simulink model "LoadFlow116BusNetwork_original"  (R2024a)
settings: Solver=FixedStepDiscrete  StartTime=0.0  StopTime=4.5  FixedStep=75e-6  RelTol=1e-3  EnableMultiTasking=on
undefined symbols (not defined in the file or in its folder): D1, D11, Delta
libraries: spsSeriesRLCBranchLib x164, spsLoadFlowBusLib x116, spsDistributedParametersLineLib x79, spsThreePhaseSeriesRLCLoadLib x60, spsThreePhaseTransformerTwoWindingsLib x52, spsThreePhaseParallelRLCLoadLib x44, spsThreePhaseVIMeasurementLib x44, spsSynchronousMachinepuStandardLib x28, spsExcitationSystemLib x28, spsHydraulicTurbineandGovernorLib x28, spsGenericPowerSystemStabilizerLib x28, spsMultiBandPowerSystemStabilizerLib x28
(part 6 of 15)

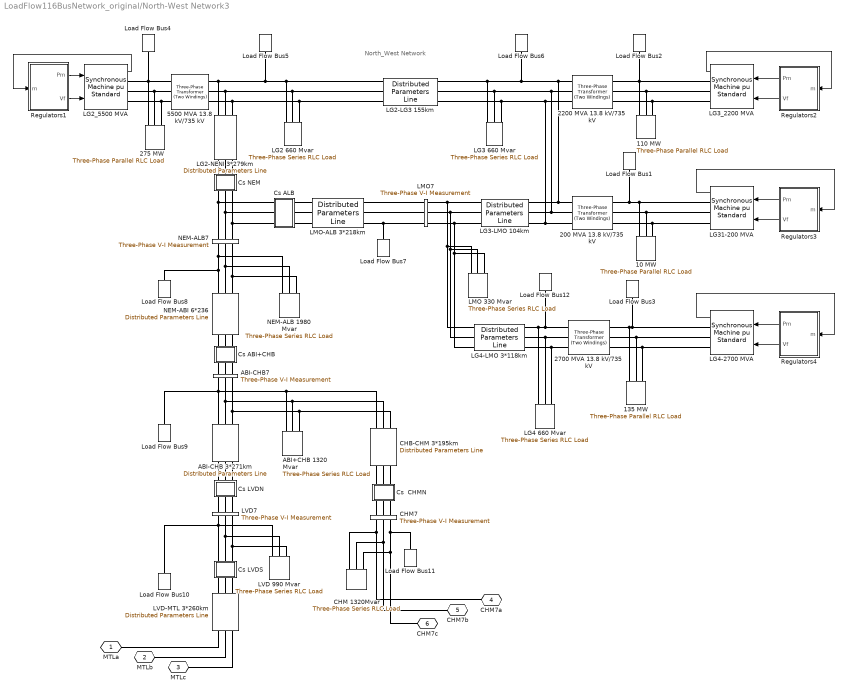
== system LoadFlow116BusNetwork_original/North-West Network3 ==
  note: North_West Network
  10 MW : spsThreePhaseParallelRLCLoadLib/Three-Phase Parallel RLC Load  LConnTagsString=A|B|C  Configuration=Y (grounded)  NominalVoltage=(13800)*1  Vabc=[1e3 1e3 1e3]  Vabcp=[1e3 1e3 1e3]  NominalFrequency=60  UnbalancedPower=off  ActivePower=10000000  InductivePower=0  CapacitivePower=0  Pabc=[10e3 9e3 11e3]  QLabc=[100 90 110]  QCabc=[100 90 110]  Pabcp=[10e3 9e3 11e3]  QLabcp=[100 90 110]  QCabcp=[100 90 110]  Measurements=None  LoadType=constant PQ
  110 MW : spsThreePhaseParallelRLCLoadLib/Three-Phase Parallel RLC Load  LConnTagsString=A|B|C  Configuration=Y (grounded)  NominalVoltage=(13800)*1  Vabc=[1e3 1e3 1e3]  Vabcp=[1e3 1e3 1e3]  NominalFrequency=60  UnbalancedPower=off  ActivePower=110000000  InductivePower=0  CapacitivePower=0  Pabc=[10e3 9e3 11e3]  QLabc=[100 90 110]  QCabc=[100 90 110]  Pabcp=[10e3 9e3 11e3]  QLabcp=[100 90 110]  QCabcp=[100 90 110]  Measurements=None  LoadType=constant PQ
  135 MW : spsThreePhaseParallelRLCLoadLib/Three-Phase Parallel RLC Load  LConnTagsString=A|B|C  Configuration=Y (grounded)  NominalVoltage=(13800)*1  Vabc=[1e3 1e3 1e3]  Vabcp=[1e3 1e3 1e3]  NominalFrequency=60  UnbalancedPower=off  ActivePower=135000000  InductivePower=0  CapacitivePower=0  Pabc=[10e3 9e3 11e3]  QLabc=[100 90 110]  QCabc=[100 90 110]  Pabcp=[10e3 9e3 11e3]  QLabcp=[100 90 110]  QCabcp=[100 90 110]  Measurements=None  LoadType=constant PQ
  200 MVA 13.8 kV/735 kV : spsThreePhaseTransformerTwoWindingsLib/Three-Phase Transformer (Two Windings)  Winding1Connection=Delta (D1)  Winding2Connection=Yg  CoreType=Three single-phase transformers  SetSaturation=off  Hysteresis=off  DataFile='basic_model'  SetInitialFlux=off  Measurements=None  UNITS=pu  NominalPower=[ 200e6 60 ]  Winding1="[ 13.8e3 0.002  0.0]"  Winding2=[ 735e3 0.002 0.12]  Rm=500  Lm=500  L0=0.5  Saturation="[ 0,0  ;  0.005,1.2  ;  1.0,1.4 ]"  InitialFluxes=[ 0.8 , -0.8 , 0.7 ]  BreakLoop=off  DiscreteSolver=Trapezoidal iterative  DataType=off  TransfoNumber=0
  2200 MVA 13.8 kV/735 kV : spsThreePhaseTransformerTwoWindingsLib/Three-Phase Transformer (Two Windings)  Winding1Connection=Delta (D1)  Winding2Connection=Yg  CoreType=Three single-phase transformers  SetSaturation=off  Hysteresis=off  DataFile='basic_model'  SetInitialFlux=off  Measurements=None  UNITS=pu  NominalPower=[ 2200e6 60 ]  Winding1="[ 13.8e3 0.002  0.0]"  Winding2=[ 735e3 0.002 0.12]  Rm=500  Lm=500  L0=0.5  Saturation="[ 0,0  ;  0.005,1.2  ;  1.0,1.4 ]"  InitialFluxes=[ 0.8 , -0.8 , 0.7 ]  BreakLoop=off  DiscreteSolver=Trapezoidal iterative  DataType=off  TransfoNumber=0
  2700 MVA 13.8 kV/735 kV : spsThreePhaseTransformerTwoWindingsLib/Three-Phase Transformer (Two Windings)  Winding1Connection=Delta (D1)  Winding2Connection=Yg  CoreType=Three single-phase transformers  SetSaturation=off  Hysteresis=off  DataFile='basic_model'  SetInitialFlux=off  Measurements=None  UNITS=pu  NominalPower=[ 2700e6 60 ]  Winding1="[ 13.8e3 0.002  0.0]"  Winding2=[ 735e3 0.002 0.12]  Rm=500  Lm=500  L0=0.5  Saturation="[ 0,0  ;  0.005,1.2  ;  1.0,1.4 ]"  InitialFluxes=[ 0.8 , -0.8 , 0.7 ]  BreakLoop=off  DiscreteSolver=Trapezoidal iterative  DataType=off  TransfoNumber=0
  275 MW : spsThreePhaseParallelRLCLoadLib/Three-Phase Parallel RLC Load  LConnTagsString=A|B|C  Configuration=Y (grounded)  NominalVoltage=(13800)*1  Vabc=[1e3 1e3 1e3]  Vabcp=[1e3 1e3 1e3]  NominalFrequency=60  UnbalancedPower=off  ActivePower=275000000  InductivePower=0  CapacitivePower=0  Pabc=[10e3 9e3 11e3]  QLabc=[100 90 110]  QCabc=[100 90 110]  Pabcp=[10e3 9e3 11e3]  QLabcp=[100 90 110]  QCabcp=[100 90 110]  Measurements=None  LoadType=constant PQ
  5500 MVA 13.8 kV/735 kV : spsThreePhaseTransformerTwoWindingsLib/Three-Phase Transformer (Two Windings)  Winding1Connection=Delta (D1)  Winding2Connection=Yg  CoreType=Three single-phase transformers  SetSaturation=off  Hysteresis=off  DataFile='basic_model'  SetInitialFlux=off  Measurements=None  UNITS=pu  NominalPower=[ 5500e6 60 ]  Winding1="[ 13.8e3 0.002  0.0]"  Winding2=[ 735e3 0.002 0.12]  Rm=500  Lm=500  L0=0.5  Saturation="[ 0,0  ;  0.005,1.2  ;  1.0,1.4 ]"  InitialFluxes=[ 0.8 , -0.8 , 0.7 ]  BreakLoop=off  DiscreteSolver=Trapezoidal iterative  DataType=off  TransfoNumber=0
  ABI+CHB 1320 Mvar : spsThreePhaseSeriesRLCLoadLib/Three-Phase Series RLC Load  LConnTagsString=A|B|C  Configuration=Y (grounded)  NominalVoltage=735e3  Vabc=[1e3 1e3 1e3]  Vabcp=[1e3 1e3 1e3]  NominalFrequency=60  UnbalancedPower=off  ActivePower=4400000  InductivePower=1320e6  CapacitivePower=0  Pabc=[10e3 9e3 11e3]  QLabc=[100 90 110]  QCabc=[100 90 110]  Pabcp=[10e3 9e3 11e3]  QLabcp=[100 90 110]  QCabcp=[100 90 110]  Measurements=None  LoadType=constant Z
  ABI-CHB 3*271km : spsDistributedParametersLineLib/Distributed Parameters Line  Phases=3  Length=271  Frequency=60  Resistance="[0.01273  0.3864]/3"  Inductance="[0.9337e-3  4.1264e-3]/3"  Capacitance=[12.74e-9 7.751e-9]*3  x1=[-0.001575 1.61368784010764e-08 -103484.456536196 -819305.84711539;-0.0015 1.60869587384057e-08 -80280.8596538857 -821903.919579448;-0.001425 1.60241794070583e-08 -57013.0874807064 -823844.974625746;-0.00135 1.5948590591871e-08 -33699.7399177245 -825127.460604578;-0.001275 1.58602527173862e-08 -10359.4532982758 -825750.352316277;-0.0012 1.57592363995491e-08 12989.1145096347 -825713.151830738;-0.001125 1.56456223892586e-08 36327.2990181464 -825015.88888546;-0.00105 1.55195015078162e-08 59636.4440396491 -823659.120861774;-0.000975 1.53809745743248e-08 82897.9166002548 -821643.932339278;-0.0009 1.52301523250955e-08 106093.121834711 -818971.934228844;-0.000825 1.50671553251267e-08 129203.517850851 -815645.262484878;-0.00075 1.48921138717261e-08 152210.630551702 -811666.576397873;-0.000675 1.47051678903535e-08 175096.068403391 -807039.05646861;-0.0006 1.45064668227659e-08 197841.537137057 -801766.401865718;-0.000525 1.42961695075566e-08 220428.854373013 -795852.827468612;-0.00045 1.40744440531817e-08 242839.964155458 -789303.060498184;-0.000375 1.38414677035769e-08 265056.951386133 -782122.336737935;-0.0003 1.35974266964714e-08 287062.056145378 -774316.396348571;-0.000225 1.33425161145124e-08 308837.687889136 -765891.479279405;-0.00015 1.30769397293187e-08 330366.439510571 -756854.320280235;-7.5e-05 1.28009098385893e-08 351631.101255038 -747212.143517692]  x2=[-0.001575 3.62536968240975e-08 -329701.158011595 -748762.187115594;-0.0015 3.6150290335032e-08 -308401.441010007 -757783.743021083;-0.001425 3.60179858569907e-08 -286855.192615176 -766199.538196882;-0.00135 3.5856889152149e-08 -265079.636568401 -774002.845185091;-0.001275 3.56671289987478e-08 -243092.179916007 -781187.426141501;-0.0012 3.54488570881504e-08 -220910.399094423 -787747.537822021;-0.001125 3.52022479035825e-08 -198552.025879845 -793677.936173748;-0.00105 3.49274985806529e-08 -176034.933213728 -798973.880526977;-0.000975 3.46248287497665e-08 -153377.120915423 -803631.137384824;-0.0009 3.42944803605553e-08 -130596.701293408 -807645.983807413;-0.000825 3.39367174884669e-08 -107711.884666575 -811015.210387945;-0.00075 3.35518261236675e-08 -84740.9648071874 -813736.123818242;-0.000675 3.31401139424249e-08 -61702.3043171127 -815806.549041739;-0.0006 3.27019100611576e-08 -38614.3199490438 -817224.83099219;-0.000525 3.22375647733433e-08 -15495.4678844266 -817989.835916705;-0.00045 3.17474492695005e-08 7635.77102012883 -818100.952282053;-0.000375 3.1231955340464e-08 30760.906006162 -817558.091263511;-0.0003 3.06914950641932e-08 53861.4511945915 -816361.686815871;-0.000225 3.01265004763637e-08 76918.9403630438 -814512.695326543;-0.00015 2.95374232250043e-08 99914.9417074692 -812012.594851034;-7.5e-05 2.89247342094566e-08 122831.072576244 -808863.383931409]  x3=[-0.001575 1.03818529884453e-10 -747.84143391774 -1501.46113433694;-0.0015 1.07871324417376e-10 -705.095036948362 -1522.00231179514;-0.001425 1.11837888264047e-10 -661.784997794763 -1541.3268238927;-0.00135 1.15715050614017e-10 -617.945937839577 -1559.41922291034;-0.001275 1.19499712123026e-10 -573.612901356573 -1576.2650460611;-0.0012 1.2318884739057e-10 -528.821327496795 -1591.8508270517;-0.001125 1.26779507378363e-10 -483.607021959054 -1606.16410684729;-0.00105 1.30268821767749e-10 -438.006128367395 -1619.193443631;-0.000975 1.33654001254194e-10 -392.055099378437 -1630.92842195037;-0.0009 1.36932339777011e-10 -345.790667541681 -1641.35966104326;-0.000825 1.40101216682546e-10 -299.249815936066 -1650.47882233677;-0.00075 1.43158098819084e-10 -252.469748606267 -1658.27861611287;-0.000675 1.4610054256182e-10 -205.48786082235 -1664.75280733577;-0.0006 1.48926195766244e-10 -158.341709186561 -1669.89622063605;-0.000525 1.5163279964842e-10 -111.068981611157 -1673.70474444782;-0.00045 1.54218190590617e-10 -63.7074671912658 -1676.17533429543;-0.000375 1.56680301870874e-10 -16.2950259968589 -1677.30601522714;-0.0003 1.59017165315103e-10 31.1304411920077 -1677.09588339392;-0.000225 1.61226912870424e-10 78.531023182497 -1675.54510677195;-0.00015 1.63307778098451e-10 125.868828674619 -1672.65492502832;-7.5e-05 1.65258097587359e-10 173.106016550957 -1668.4276485301]  x4=[-0.001575 9.2267726494399e-11 -7080.29438162533 -14859.1258761631;-0.0015 8.935033754735e-11 -6657.38891400197 -15053.3510061735;-0.001425 8.63615233075717e-11 -6229.16163154223 -15235.5427177136;-0.00135 8.33036729874369e-11 -5795.95485258361 -15405.5553695168;-0.001275 8.01792309857049e-11 -5358.11487599691 -15563.2530560704;-0.0012 7.69906949335063e-11 -4915.99170436025 -15708.5097162568;-0.001125 7.3740613697775e-11 -4469.93876417232 -15841.2092341243;-0.00105 7.0431585343723e-11 -4020.31262332866 -15961.2455317087;-0.000975 6.70662550579865e-11 -3567.47270608676 -16068.5226538302;-0.0009 6.36473130341048e-11 -3111.78100574778 -16162.9548447989;-0.000825 6.01774923220202e-11 -2653.60179528465 -16244.4666169662;-0.00075 5.66595666433199e-11 -2193.30133614784 -16312.9928110686;-0.000675 5.30963481739653e-11 -1731.24758548155 -16368.4786483149;-0.0006 4.94906852962818e-11 -1267.8099019844 -16410.8797741759;-0.000525 4.58454603220054e-11 -803.358750649743 -16440.1622938403;-0.00045 4.21635871882066e-11 -338.26540662162 -16456.30279931;-0.000375 3.84480091279341e-11 127.098341596922 -16459.2883881117;-0.0003 3.4701696317439e-11 592.360489345862 -16449.1166736115;-0.000225 3.09276435018615e-11 1057.14911318304 -16425.7957869224;-0.00015 2.71288676012774e-11 1521.09266819406 -16389.3443704043;-7.5e-05 2.33084052990185e-11 1983.82028499962 -16339.7915627619]  x5=0.00153261764655846  V1=ones(3,3)  V2=ones(3,3)  I1=ones(3,3)  I2=ones(3,3)  nHarmo=1  Measurements=None  Decoupling=off  VsMag0=[ 1 1 1]  VrMag0=[ 1 1 1]  VsAngle0=[0 -120 120]  VrAngle0=[0 -120 120]  IsMag0=[ 1 1 1]  IrMag0=[ 1 1 1]  IsAngle0=[0 -120 120]  IrAngle0=[0 -120 120]
      settings: AttributesFormatString=\n  LibrarySourceBlock=sps_lib/Power Grid Elements/Distributed Parameters Line
  ABI-CHB7 : spsThreePhaseVIMeasurementLib/Three-Phase V-I Measurement  VoltageMeasurement=no  SetLabelV=on  LabelV=Vabc_ABI7  Vpu=on  VpuLL=off  CurrentMeasurement=no  SetLabelI=off  LabelI=A1  Ipu=off  Pbase=100e6  Vbase=500e3  OutputType=Magnitude  PhasorSimulation=off  PSBequivalent=0
  CHB-CHM 3*195km : spsDistributedParametersLineLib/Distributed Parameters Line  Phases=3  Length=195  Frequency=60  Resistance="[0.01273  0.3864]/3"  Inductance="[0.9337e-3  4.1264e-3]/3"  Capacitance=[12.74e-9 7.751e-9]*3  x1=[-0.001125 1.56456223892586e-08 0 0;-0.00105 1.55195015078162e-08 0 0;-0.000975 1.53809745743248e-08 0 0;-0.0009 1.52301523250955e-08 0 0;-0.000825 1.50671553251267e-08 0 0;-0.00075 1.48921138717261e-08 0 0;-0.000675 1.47051678903535e-08 175096.068403391 -807039.05646861;-0.0006 1.45064668227659e-08 197841.537137057 -801766.401865718;-0.000525 1.42961695075566e-08 220428.854373013 -795852.827468612;-0.00045 1.40744440531817e-08 242839.964155458 -789303.060498184;-0.000375 1.38414677035769e-08 265056.951386133 -782122.336737935;-0.0003 1.35974266964714e-08 287062.056145378 -774316.396348571;-0.000225 1.33425161145124e-08 308837.687889136 -765891.479279405;-0.00015 1.30769397293187e-08 330366.439510571 -756854.320280235;-7.5e-05 1.28009098385893e-08 351631.101255038 -747212.143517692]  x2=[-0.001125 1.08131047076709e-08 0 0;-0.00105 1.07075759161992e-08 0 0;-0.000975 1.05934876523715e-08 0 0;-0.0009 1.04709311166003e-08 0 0;-0.000825 1.03400042787051e-08 0 0;-0.00075 1.02008117995969e-08 0 0;-0.000675 1.00534649476137e-08 86661.6913680983 -814290.344127133;-0.0006 9.89808150957456e-09 109647.510746662 -811514.902082533;-0.000525 9.7347856966224e-09 132545.679582797 -808090.747441803;-0.00045 9.56370804493158e-09 155337.893430691 -804020.617421771;-0.000375 9.38498531135928e-09 178005.932543326 -799307.7656221;-0.0003 9.19876036412418e-09 200531.676437068 -793955.959424409;-0.000225 9.00518206859974e-09 222897.118376904 -787969.476980688;-0.00015 8.80440516831357e-09 245084.37977075 -781353.103793406;-7.5e-05 8.59659016124777e-09 267075.724461323 -774112.128890055]  x3=[-0.001125 4.4858512859097e-11 0 0;-0.00105 4.35746292342984e-11 0 0;-0.000975 4.2255912717604e-11 0 0;-0.0009 4.09034174708204e-11 0 0;-0.000825 3.95182246579538e-11 0 0;-0.00075 3.81014415809448e-11 0 0;-0.000675 3.66542007945076e-11 335.259499976357 -5255.1630322499;-0.0006 3.51776592007834e-11 483.692851575988 -5243.58412650668;-0.000525 3.36729971245303e-11 631.739546510818 -5227.81357984227;-0.00045 3.21414173695899e-11 779.281238518107 -5207.86399899035;-0.000375 3.05841442573845e-11 926.199985026726 -5183.75133134064;-0.0003 2.90024226482128e-11 1072.37834143865 -5155.4948521907;-0.000225 2.73975169461281e-11 1217.69945501237 -5123.11714933764;-0.00015 2.57707100881928e-11 1362.04715827318 -5086.64410502172;-7.5e-05 2.4123302518918e-11 1505.30606187568 -5046.10487523651]  x4=[-0.001125 6.43220354740688e-11 0 0;-0.00105 6.53718926848705e-11 0 0;-0.000975 6.63694926048834e-11 0 0;-0.0009 6.73140377679952e-11 0 0;-0.000825 6.82047731192546e-11 0 0;-0.00075 6.90409866184505e-11 0 0;-0.000675 6.98220098093062e-11 265.942029613462 -12956.0177279471;-0.0006 7.05472183538328e-11 632.108856780861 -12943.3211843326;-0.000525 7.12160325314161e-11 997.770385799739 -12920.2779478029;-0.00045 7.18279177022355e-11 1362.63431243861 -12886.9064387685;-0.000375 7.23823847346478e-11 1726.40897005712 -12843.2333339032;-0.0003 7.28789903961908e-11 2088.80356275991 -12789.2935448189;-0.000225 7.33173377078971e-11 2449.52839785439 -12725.1301901576;-0.00015 7.36970762616325e-11 2808.29511742667 -12650.7945611234;-7.5e-05 7.40179025002075e-11 3164.81692885044 -12566.3460804806]  x5=0.0011028060556417  V1=ones(3,3)  V2=ones(3,3)  I1=ones(3,3)  I2=ones(3,3)  nHarmo=1  Measurements=None  Decoupling=off  VsMag0=[ 1 1 1]  VrMag0=[ 1 1 1]  VsAngle0=[0 -120 120]  VrAngle0=[0 -120 120]  IsMag0=[ 1 1 1]  IrMag0=[ 1 1 1]  IsAngle0=[0 -120 120]  IrAngle0=[0 -120 120]
      settings: AttributesFormatString=\n  LibrarySourceBlock=sps_lib/Power Grid Elements/Distributed Parameters Line
  CHM 1320Mvar : spsThreePhaseSeriesRLCLoadLib/Three-Phase Series RLC Load  LConnTagsString=A|B|C  Configuration=Y (grounded)  NominalVoltage=735e3  Vabc=[1e3 1e3 1e3]  Vabcp=[1e3 1e3 1e3]  NominalFrequency=60  UnbalancedPower=off  ActivePower=4400000  InductivePower=1320e6  CapacitivePower=0  Pabc=[10e3 9e3 11e3]  QLabc=[100 90 110]  QCabc=[100 90 110]  Pabcp=[10e3 9e3 11e3]  QLabcp=[100 90 110]  QCabcp=[100 90 110]  Measurements=None  LoadType=constant Z
  CHM7 : spsThreePhaseVIMeasurementLib/Three-Phase V-I Measurement  VoltageMeasurement=no  SetLabelV=on  LabelV=Vabc_CHM7  Vpu=on  VpuLL=off  CurrentMeasurement=no  SetLabelI=off  LabelI=A1  Ipu=off  Pbase=100e6  Vbase=735e3  OutputType=Magnitude  PhasorSimulation=off  PSBequivalent=0
  "Cs  CHMN " : Subsystem  mask{Xc=25/3}
      mask prompts: Xc "Condensator Reactance at  60Hz  (ohm):"
      mask help: Series Compensation
      mask init:
      | Cs=1/Xc/(2*pi*60);
      mask Display: disp('Cs')
  "Cs ABI+CHB " : Subsystem  mask{Xc=25/6}
      mask prompts: Xc "Condensator Reactance at  60Hz  (ohm):"
      mask help: Series Compensation
      mask init:
      | Cs=1/Xc/(2*pi*60);
      mask Display: disp('Cs')
  Cs ALB : Subsystem  mask{Xc=16/3}
      mask prompts: Xc "Reactance @ 60Hz du condensateur (ohm):"
      mask init:
      | Cs=1/Xc/(2*pi*60);
      mask Display: disp('Cs')
  "Cs LVDN " : Subsystem  mask{Xc=34/3}
      mask prompts: Xc "Condensator Reactance at  60Hz  (ohm):"
      mask help: Series Compensation
      mask init:
      | Cs=1/Xc/(2*pi*60);
      mask Display: disp('Cs')
  "Cs LVDS " : Subsystem  mask{Xc=34/3}
      mask prompts: Xc "Condensator Reactance at  60Hz  (ohm):"
      mask help: Series Compensation
      mask init:
      | Cs=1/Xc/(2*pi*60);
      mask Display: disp('Cs')
  "Cs NEM " : Subsystem  mask{Xc=16/3}
      mask prompts: Xc "Condensator Reactance at  60Hz  (ohm):"
      mask help: Series Compensation
      mask init:
      | Cs=1/Xc/(2*pi*60);
      mask Display: disp('Cs')
  LG2 660 Mvar : spsThreePhaseSeriesRLCLoadLib/Three-Phase Series RLC Load  LConnTagsString=A|B|C  Configuration=Y (grounded)  NominalVoltage=735e3  Vabc=[1e3 1e3 1e3]  Vabcp=[1e3 1e3 1e3]  NominalFrequency=60  UnbalancedPower=off  ActivePower=2200000  InductivePower=660e6  CapacitivePower=0  Pabc=[10e3 9e3 11e3]  QLabc=[100 90 110]  QCabc=[100 90 110]  Pabcp=[10e3 9e3 11e3]  QLabcp=[100 90 110]  QCabcp=[100 90 110]  Measurements=None  LoadType=constant Z
  LG2-LG3 155km : spsDistributedParametersLineLib/Distributed Parameters Line  Phases=3  Length=155  Frequency=60  Resistance="[0.01273  0.3864]"  Inductance="[0.9337e-3  4.1264e-3]"  Capacitance=[12.74e-9 7.751e-9]  x1=[-0.0009 -7.39389899420552e-10 371984.249881772 -674633.962928029;-0.000825 -7.04590728695761e-10 390907.835511709 -663848.049238342;-0.00075 -6.69228318923049e-10 409518.935399028 -652531.46557531;-0.000675 -6.33330938271727e-10 427802.672115239 -640693.258242764;-0.0006 -5.9692728255864e-10 445744.429920962 -628342.890522514;-0.000525 -5.60046452309168e-10 463329.866449524 -615490.235109549;-0.00045 -5.22717929494719e-10 480544.924172032 -602145.566219953;-0.000375 -4.84971553965284e-10 497375.84163474 -588319.551377858;-0.0003 -4.46837499595923e-10 513809.164459751 -574023.242887982;-0.000225 -4.08346250166227e-10 529831.756100236 -559268.069000591;-0.00015 -3.69528574992056e-10 545430.808341593 -544065.82477593;-7.5e-05 -3.30415504329014e-10 560593.851540132 -528428.662655429]  x2=[-0.0009 4.61714864410203e-10 375373.731714381 -666225.896356526;-0.000825 4.29491228010982e-10 394058.262242319 -655347.523812814;-0.00075 3.96924262895526e-10 412427.788624714 -643945.27648572;-0.000675 3.64040002597455e-10 430467.626543239 -632028.269157297;-0.0006 3.30864734291308e-10 448163.355227482 -619606.028100866;-0.000525 2.97424977778967e-10 465500.828982684 -606688.483465861;-0.00045 2.63747464290145e-10 482466.1884976 -593285.961339819;-0.000375 2.29859115113841e-10 499045.871923411 -579409.175493861;-0.0003 1.95787020077878e-10 515226.625714864 -565069.218818271;-0.000225 1.61558415893706e-10 530995.515224952 -550277.554455007;-0.00015 1.27200664383795e-10 546339.935044673 -535046.006634241;-7.5e-05 9.27412306090115e-11 561247.619079601 -519386.751222249]  x3=[-0.0009 7.94100563228245e-12 1272.11889165564 -2673.50704029644;-0.000825 8.04323545901243e-12 1347.19195646262 -2636.4747108115;-0.00075 8.1390356463821e-12 1421.18809663233 -2597.33482378215;-0.000675 8.22832961318747e-12 1494.0481607825 -2556.11866703523;-0.0006 8.31104597919773e-12 1565.71390569265 -2512.85918813581;-0.000525 8.38711862221548e-12 1636.12804286281 -2467.59096804942;-0.00045 8.45648673093385e-12 1705.23428430911 -2420.35019349859;-0.000375 8.5190948535481e-12 1772.97738755949 -2371.17462803567;-0.0003 8.57489294208295e-12 1839.30319981371 -2320.10358185529;-0.000225 8.62383639240016e-12 1904.15870123229 -2267.17788037035;-0.00015 8.6658860798544e-12 1967.49204731971 -2212.43983157682;-7.5e-05 8.70100839056891e-12 2029.25261036814 -2155.9331922334]  x4=[-0.0009 -9.40573285747566e-12 974.452643997522 -2530.47846704044;-0.000825 -9.48273734080599e-12 1045.60107405589 -2501.91852232137;-0.00075 -9.55216146899682e-12 1115.91366661389 -2471.3585822162;-0.000675 -9.6139497454623e-12 1185.33421486085 -2438.82307587346;-0.0006 -9.66805277759963e-12 1253.80722507267 -2404.33801167911;-0.000525 -9.71442731627271e-12 1321.27796097266 -2367.93095646583;-0.00045 -9.75303629038488e-12 1387.69248748688 -2329.63101347651;-0.000375 -9.78384883651299e-12 1452.99771385901 -2289.46879909957;-0.0003 -9.80684032357909e-12 1517.14143609029 -2247.47641839467;-0.000225 -9.8219923725402e-12 1580.07237867061 -2203.68743942845;-0.00015 -9.82929287108024e-12 1641.74023556733 -2158.13686644071;-7.5e-05 -9.82873598329235e-12 1702.09571043921 -2110.86111186252]  x5=0.000876589428843401  V1=ones(3,3)  V2=ones(3,3)  I1=ones(3,3)  I2=ones(3,3)  nHarmo=1  Measurements=None  Decoupling=off  VsMag0=[ 1 1 1]  VrMag0=[ 1 1 1]  VsAngle0=[0 -120 120]  VrAngle0=[0 -120 120]  IsMag0=[ 1 1 1]  IrMag0=[ 1 1 1]  IsAngle0=[0 -120 120]  IrAngle0=[0 -120 120]
      settings: AttributesFormatString=\n  LibrarySourceBlock=sps_lib/Power Grid Elements/Distributed Parameters Line
  LG2-NENI 3*279km : spsDistributedParametersLineLib/Distributed Parameters Line  Phases=3  Length=279  Frequency=60  Resistance="[0.01273  0.3864]/3"  Inductance="[0.9337e-3  4.1264e-3]/3"  Capacitance=[12.74e-9 7.751e-9]*3  x1=[-0.00165 -1.05053432834168e-09 168997.444323887 -751627.644710067;-0.001575 -1.0228125511771e-09 190178.800706938 -746549.517209643;-0.0015 -9.94273153308662e-10 211208.131066537 -740874.609447753;-0.001425 -9.64938948694363e-10 232068.624877755 -734607.457858831;-0.00135 -9.34833386648538e-10 252743.606581014 -727753.072307968;-0.001275 -9.03980533096857e-10 273216.548912279 -720316.932086098;-0.0012 -8.72405051338384e-10 293471.086114697 -712304.981529936;-0.001125 -8.40132182330116e-10 313491.027021134 -703723.625270172;-0.00105 -8.07187724509747e-10 333260.367997143 -694579.723111699;-0.000975 -7.73598013172791e-10 352763.305734029 -684880.584549996;-0.0009 -7.39389899420552e-10 371984.249881772 -674633.962928028;-0.000825 -7.0459072869576e-10 390907.835511709 -663848.049238342;-0.00075 -6.69228318923049e-10 409518.935399028 -652531.46557531;-0.000675 -6.33330938271727e-10 427802.672115239 -640693.258242764;-0.0006 -5.9692728255864e-10 445744.429920962 -628342.890522514;-0.000525 -5.60046452309168e-10 463329.866449524 -615490.235109549;-0.00045 -5.22717929494719e-10 480544.924172032 -602145.566219953;-0.000375 -4.84971553965284e-10 497375.84163474 -588319.551377858;-0.0003 -4.46837499595923e-10 513809.164459751 -574023.242887982;-0.000225 -4.08346250166227e-10 529831.756100236 -559268.069000591;-0.00015 -3.69528574992056e-10 545430.808341593 -544065.82477593;-7.5e-05 -3.30415504329014e-10 560593.851540132 -528428.662655429]  x2=[-0.00165 9.46370688349288e-09 -47534.306464739 -809002.983106157;-0.001575 9.44825499220037e-09 -24644.3461225168 -810023.426229689;-0.0015 9.42525031043025e-09 -1734.68546707527 -810396.349020067;-0.001425 9.39471122777314e-09 21176.361869387 -810121.453368519;-0.00135 9.35666215670445e-09 44070.4811461802 -809198.959022422;-0.001275 9.31113351306941e-09 66929.371154646 -807629.603409641;-0.0012 9.25816169176916e-09 89734.7588478645 -805414.641049042;-0.001125 9.19778903766712e-09 112468.413947848 -802555.842547646;-0.00105 9.13006381173927e-09 135112.163518546 -799055.493185233;-0.000975 9.05504015249497e-09 157647.906493013 -794916.391087527;-0.0009 8.97277803269953e-09 180057.628143123 -790141.844989414;-0.000825 8.88334321143286e-09 202323.414480269 -784735.671589993;-0.00075 8.78680718152267e-09 224427.466575532 -778702.19250156;-0.000675 8.68324711239424e-09 246352.11478787 -772046.230794985;-0.0006 8.57274578838229e-09 268079.83288896 -764773.107144217;-0.000525 8.45539154255452e-09 289593.252073398 -756888.635573017;-0.00045 8.33127818609946e-09 310875.174843053 -748399.118807326;-0.000375 8.20050493333526e-09 331908.588754489 -739311.34323695;-0.0003 8.06317632239929e-09 352676.680018446 -729632.573490633;-0.000225 7.91940213168192e-09 373162.846940531 -719370.546628821;-0.00015 7.76929729207141e-09 393350.713192354 -708533.465958772;-7.5e-05 7.61298179507985e-09 413224.140902519 -697129.994476961]  x3=[-0.00165 2.19858422182134e-11 -1677.04894976931 -1941.35400834169;-0.001575 2.39277038246712e-11 -1621.49508617303 -1987.98793711278;-0.0015 2.58504379907977e-11 -1564.64502421457 -2033.03269874418;-0.001425 2.77525077123194e-11 -1506.54420896362 -2076.45228514265;-0.00135 2.96323925038034e-11 -1447.23908532292 -2118.21198735516;-0.001275 3.14885896141107e-11 -1386.77706090092 -2158.27842331471;-0.0012 3.3319615227672e-11 -1325.20646811483 -2196.61956452543;-0.001125 3.51240056506276e-11 -1262.57652555448 -2233.20476166568;-0.00105 3.69003184808813e-11 -1198.93729863766 -2268.00476908862;-0.000975 3.86471337611353e-11 -1134.33965958867 -2300.9917682008;-0.0009 4.03630551139815e-11 -1068.83524677178 -2332.13938969983;-0.000825 4.20467108581451e-11 -1002.47642341235 -2361.42273465366;-0.00075 4.36967551049849e-11 -935.316235738447 -2388.81839440439;-0.000675 4.53118688343766e-11 -867.408370576513 -2414.30446928078;-0.0006 4.6890760949117e-11 -798.807112434934 -2437.86058610452;-0.000525 4.84321693070073e-11 -729.567300109833 -2459.46791447625;-0.00045 4.99348617297906e-11 -659.744282847778 -2479.10918182827;-0.000375 5.13976369881361e-11 -589.393876100441 -2496.76868723197;-0.0003 5.28193257618836e-11 -518.572316906578 -2512.43231394895;-0.000225 5.41987915747797e-11 -447.336218937002 -2526.08754071566;-0.00015 5.55349317029603e-11 -375.742527238481 -2537.72345175276;-7.5e-05 5.68266780564506e-11 -303.84847271274 -2547.33074549099]  x4=[-0.00165 7.86236789415688e-12 -141.249463962095 -15427.0315937077;-0.001575 6.19679283700467e-12 294.936850751302 -15424.8591939197;-0.0015 4.52626415847266e-12 730.887397458894 -15410.3563977004;-0.001425 2.85211725362654e-12 1166.25368396391 -15383.5347983631;-0.00135 1.17569040988672e-12 1600.68768511825 -15344.415836684;-0.001275 -5.01676262778087e-13 2033.84212102844 -15293.0307837624;-0.0012 -2.17864190311434e-12 2465.37073466591 -15229.4207160235;-0.001125 -3.85386597044758e-12 2894.92856865953 -15153.6364823822;-0.00105 -5.52600931629018e-12 3322.17224104926 -15065.7386635953;-0.000975 -7.19373525483611e-12 3746.76021978042 -14965.7975238342;-0.0009 -8.85571063148715e-12 4168.35309571925 -14853.892954517;-0.000825 -1.05106068885563e-11 4586.61385397131 -14730.1144104441;-0.00075 -1.21571011272964e-11 5001.20814328604 -14594.5608382898;-0.000675 -1.37938771654053e-11 5411.80454333208 -14447.3405975056;-0.0006 -1.54196265891615e-11 5818.07482962957 -14288.5713736996;-0.000525 -1.70330497993505e-11 6219.69423592778 -14118.3800845598;-0.00045 -1.86328570501444e-11 6616.3417138183 -13936.9027783989;-0.000375 -2.02177694801046e-11 7007.70018937623 -13744.2845253988;-0.0003 -2.17865201344847e-11 7393.45681662417 -13540.6793016436;-0.000225 -2.33378549780142e-11 7773.30322761658 -13326.2498660341;-0.00015 -2.48705338973555e-11 8146.93577894437 -13101.1676301801;-7.5e-05 -2.63833316924311e-11 8514.05579446277 -12865.6125213771]  x5=0.00157786097191812  V1=ones(3,3)  V2=ones(3,3)  I1=ones(3,3)  I2=ones(3,3)  nHarmo=1  Measurements=None  Decoupling=off  VsMag0=[ 1 1 1]  VrMag0=[ 1 1 1]  VsAngle0=[0 -120 120]  VrAngle0=[0 -120 120]  IsMag0=[ 1 1 1]  IrMag0=[ 1 1 1]  IsAngle0=[0 -120 120]  IrAngle0=[0 -120 120]
      settings: AttributesFormatString=\n  LibrarySourceBlock=sps_lib/Power Grid Elements/Distributed Parameters Line
  LG2_5500 MVA : spsSynchronousMachinepuStandardLib/Synchronous Machine pu Standard  PresetModel=No  MechanicalLoad=Mechanical power Pm  ShowDetailedParameters=on  RotorType=Salient-pole  Units=per unit standard parameters  MeasurementBus=off  NominalParameters="[5500E6  13800   60 ]"  Reactances1=[ 31 32 33 34 35 36 37 ]  Reactances2=[ 1.305, 0.296, 0.252, 0.474, 0.243, 0.18 ]  dAxisTimeConstants=Short-circuit  qAxisTimeConstants=Open-circuit  TimeConstants1=[]  TimeConstants2=[]  TimeConstants3=[]  TimeConstants4=[]  TimeConstants5=[ 1.01, 0.053, 0.1 ]  TimeConstants6=[]  TimeConstants7=[]  TimeConstants8=[]  StatorResistance=2.8544e-3  Mechanical="[ 4.1  0  32]"  PolePairs=32  InitialConditions=[0 -65.2434 0.985682 0.985682 0.985682 -1.22427 -121.224 118.776 1.47412]  SetSaturation=off  Saturation=[0.6404,0.7127,0.8441,0.9214,0.9956,1.082,1.19,1.316,1.457;0.7,0.7698,0.8872,0.9466,0.9969,1.046,1.1,1.151,1.201]  LoadFlowParameters=[2 4000000000 0 0 0]  TsPowergui=0  TsBlock=-1  IterativeModel=Trapezoidal non iterative  IterativeDiscreteModel=Trapezoidal non iterative  BusType=swing  Pref=0  Qref=0  Qmin=-Inf  Qmax=Inf  PLF=0  QLF=0
  LG3 660 Mvar : spsThreePhaseSeriesRLCLoadLib/Three-Phase Series RLC Load  LConnTagsString=A|B|C  Configuration=Y (grounded)  NominalVoltage=735e3  Vabc=[1e3 1e3 1e3]  Vabcp=[1e3 1e3 1e3]  NominalFrequency=60  UnbalancedPower=off  ActivePower=2200000  InductivePower=660e6  CapacitivePower=0  Pabc=[10e3 9e3 11e3]  QLabc=[100 90 110]  QCabc=[100 90 110]  Pabcp=[10e3 9e3 11e3]  QLabcp=[100 90 110]  QCabcp=[100 90 110]  Measurements=None  LoadType=constant Z
  LG3-LMO 104km : spsDistributedParametersLineLib/Distributed Parameters Line  Phases=3  Length=104  Frequency=60  Resistance="[0.01273  0.3864]"  Inductance="[0.9337e-3  4.1264e-3]"  Capacitance=[12.74e-9 7.751e-9]  x1=[-0.0006 3.30864734291307e-10 0 0;-0.000525 2.97424977778967e-10 0 0;-0.00045 2.63747464290145e-10 0 0;-0.000375 2.29859115113841e-10 499045.871923411 -579409.175493861;-0.0003 1.95787020077878e-10 515226.625714864 -565069.218818271;-0.000225 1.61558415893706e-10 530995.515224952 -550277.554455007;-0.00015 1.27200664383795e-10 546339.935044673 -535046.006634241;-7.5e-05 9.27412306090115e-11 561247.619079601 -519386.751222249]  x2=[-0.0006 2.62550128158576e-09 0 0;-0.000525 2.58074460401706e-09 0 0;-0.00045 2.53392491869863e-09 0 0;-0.000375 2.48507965257055e-09 445735.713706799 -651849.764162571;-0.0003 2.43424785179119e-09 463985.717973745 -638987.984734666;-0.000225 2.38147015052435e-09 481864.819156963 -625615.408088608;-0.00015 2.3267887384569e-09 499358.724976525 -611742.72405756;-7.5e-05 2.27024732707299e-09 516453.451071785 -597381.022252878]  x3=[-0.0006 7.53971500699014e-12 0 0;-0.000525 7.8861425677903e-12 0 0;-0.00045 8.22626606688381e-12 0 0;-0.000375 8.55981361474953e-12 -337.815764584387 -872.913223710706;-0.0003 8.88651857858117e-12 -313.00240355855 -882.114195188783;-0.000225 9.20611979542938e-12 -287.938833200407 -890.610018076025;-0.00015 9.51836178097149e-12 -262.645088944615 -898.393900941608;-7.5e-05 9.8229949337417e-12 -237.141390223325 -905.459621468666]  x4=[-0.0006 -8.197747487121e-13 0 0;-0.000525 -1.16487248924766e-12 0 0;-0.00045 -1.50903904853847e-12 0 0;-0.000375 -1.85199930510295e-12 3507.69484614604 -3894.26054707351;-0.0003 -2.19347910175946e-12 3616.38515846589 -3793.53952688912;-0.000225 -2.53320546478339e-12 3722.1845878226 -3689.78600925004;-0.00015 -2.87090682211811e-12 3825.00855977115 -3583.08293313079;-7.5e-05 -3.20631322046557e-12 3924.77487840161 -3473.5155953378]  x5=0.000588163229675572  V1=ones(3,3)  V2=ones(3,3)  I1=ones(3,3)  I2=ones(3,3)  nHarmo=1  Measurements=None  Decoupling=off  VsMag0=[ 1 1 1]  VrMag0=[ 1 1 1]  VsAngle0=[0 -120 120]  VrAngle0=[0 -120 120]  IsMag0=[ 1 1 1]  IrMag0=[ 1 1 1]  IsAngle0=[0 -120 120]  IrAngle0=[0 -120 120]
      settings: AttributesFormatString=\n  LibrarySourceBlock=sps_lib/Power Grid Elements/Distributed Parameters Line
  LG31-200 MVA : spsSynchronousMachinepuStandardLib/Synchronous Machine pu Standard  PresetModel=No  MechanicalLoad=Mechanical power Pm  ShowDetailedParameters=on  RotorType=Salient-pole  Units=per unit standard parameters  MeasurementBus=off  NominalParameters="[200E6  13800   60 ]"  Reactances1=[ 31 32 33 34 35 36 37 ]  Reactances2=[ 1.305, 0.296, 0.252, 0.474, 0.243, 0.18 ]  dAxisTimeConstants=Short-circuit  qAxisTimeConstants=Open-circuit  TimeConstants1=[]  TimeConstants2=[]  TimeConstants3=[]  TimeConstants4=[]  TimeConstants5=[ 1.01, 0.053, 0.1 ]  TimeConstants6=[]  TimeConstants7=[]  TimeConstants8=[]  StatorResistance=2.8544e-3  Mechanical="[ 3.2  0  32]"  PolePairs=32  InitialConditions=[0 -67.6291 0.902477 0.902477 0.902477 -4.2812 -124.281 115.719 1.45511]  SetSaturation=off  Saturation=[0.6404,0.7127,0.8441,0.9214,0.9956,1.082,1.19,1.316,1.457;0.7,0.7698,0.8872,0.9466,0.9969,1.046,1.1,1.151,1.201]  LoadFlowParameters=[1 180000000 0 0 0]  TsPowergui=0  TsBlock=-1  IterativeModel=Trapezoidal non iterative  IterativeDiscreteModel=Trapezoidal non iterative  BusType=PV  Pref=180000000  Qref=0  Qmin=-Inf  Qmax=Inf  PLF=0  QLF=0
  LG3_2200 MVA : spsSynchronousMachinepuStandardLib/Synchronous Machine pu Standard  PresetModel=No  MechanicalLoad=Mechanical power Pm  ShowDetailedParameters=on  RotorType=Salient-pole  Units=per unit standard parameters  MeasurementBus=off  NominalParameters="[2200E6  13800   60 ]"  Reactances1=[ 31 32 33 34 35 36 37 ]  Reactances2=[ 1.305, 0.296, 0.252, 0.474, 0.243, 0.18 ]  dAxisTimeConstants=Short-circuit  qAxisTimeConstants=Open-circuit  TimeConstants1=[]  TimeConstants2=[]  TimeConstants3=[]  TimeConstants4=[]  TimeConstants5=[ 1.01, 0.053, 0.1 ]  TimeConstants6=[]  TimeConstants7=[]  TimeConstants8=[]  StatorResistance=2.8544e-3  Mechanical="[ 3.2  0  32]"  PolePairs=32  InitialConditions=[0 -70.0065 0.820496 0.820496 0.820496 -4.90643 -124.906 115.094 1.38903]  SetSaturation=off  Saturation=[0.6404,0.7127,0.8441,0.9214,0.9956,1.082,1.19,1.316,1.457;0.7,0.7698,0.8872,0.9466,0.9969,1.046,1.1,1.151,1.201]  LoadFlowParameters=[1 1800000000 0 0 0]  TsPowergui=0  TsBlock=-1  IterativeModel=Trapezoidal non iterative  IterativeDiscreteModel=Trapezoidal non iterative  BusType=PV  Pref=1800000000  Qref=0  Qmin=-Inf  Qmax=Inf  PLF=0  QLF=0
  LG4 660 Mvar : spsThreePhaseSeriesRLCLoadLib/Three-Phase Series RLC Load  LConnTagsString=A|B|C  Configuration=Y (grounded)  NominalVoltage=735e3  Vabc=[1e3 1e3 1e3]  Vabcp=[1e3 1e3 1e3]  NominalFrequency=60  UnbalancedPower=off  ActivePower=2200000  InductivePower=660e6  CapacitivePower=0  Pabc=[10e3 9e3 11e3]  QLabc=[100 90 110]  QCabc=[100 90 110]  Pabcp=[10e3 9e3 11e3]  QLabcp=[100 90 110]  QCabcp=[100 90 110]  Measurements=None  LoadType=constant Z
  LG4-2700 MVA : spsSynchronousMachinepuStandardLib/Synchronous Machine pu Standard  PresetModel=No  MechanicalLoad=Mechanical power Pm  ShowDetailedParameters=on  RotorType=Salient-pole  Units=per unit standard parameters  MeasurementBus=off  NominalParameters="[2700E6  13800   60 ]"  Reactances1=[ 31 32 33 34 35 36 37 ]  Reactances2=[ 1.305, 0.296, 0.252, 0.474, 0.243, 0.18 ]  dAxisTimeConstants=Short-circuit  qAxisTimeConstants=Open-circuit  TimeConstants1=[]  TimeConstants2=[]  TimeConstants3=[]  TimeConstants4=[]  TimeConstants5=[ 1.01, 0.053, 0.1 ]  TimeConstants6=[]  TimeConstants7=[]  TimeConstants8=[]  StatorResistance=2.8544e-3  Mechanical="[ 3.7  0  32]"  PolePairs=32  InitialConditions=[0 -69.506 0.926038 0.926038 0.926038 -2.40174 -122.402 117.598 1.38766]  SetSaturation=off  Saturation=[0.6404,0.7127,0.8441,0.9214,0.9956,1.082,1.19,1.316,1.457;0.7,0.7698,0.8872,0.9466,0.9969,1.046,1.1,1.151,1.201]  LoadFlowParameters=[1 2500000000 0 0 0]  TsPowergui=0  TsBlock=-1  IterativeModel=Trapezoidal non iterative  IterativeDiscreteModel=Trapezoidal non iterative  BusType=PV  Pref=2500000000  Qref=0  Qmin=-Inf  Qmax=Inf  PLF=0  QLF=0
  LG4-LMO 3*118km : spsDistributedParametersLineLib/Distributed Parameters Line  Phases=3  Length=118  Frequency=60  Resistance="[0.01273  0.3864]/3"  Inductance="[0.9337e-3  4.1264e-3]/3"  Capacitance=[12.74e-9 7.751e-9]*3  x1=[-0.000675 -1.14792243718871e-10 400494.98918032 -665247.597360336;-0.0006 -1.51297168687587e-10 419141.837998181 -653659.450927146;-0.000525 -1.87681149014578e-10 437453.631243831 -641548.77913021;-0.00045 -2.23915099902665e-10 455415.73074993 -628925.263055263;-0.000375 -2.59970056485905e-10 473013.777888962 -615798.993747908;-0.0003 -2.95817196983666e-10 490233.705051303 -602180.464146992;-0.000225 -3.31427865740313e-10 507061.746890653 -588080.560696707;-0.00015 -3.66773596132104e-10 523484.451327844 -573510.554644136;-7.5e-05 -4.01826133322971e-10 539488.690304224 -558482.093029187]  x2=[-0.000675 2.66815917360147e-09 369322.642211784 -697989.574610583;-0.0006 2.62550128158576e-09 388907.582416659 -687269.594638257;-0.000525 2.58074460401706e-09 408181.635850635 -676000.221867554;-0.00045 2.53392491869863e-09 427129.395130302 -664190.464862641;-0.000375 2.48507965257055e-09 445735.713706799 -651849.764162571;-0.0003 2.43424785179119e-09 463985.717973745 -638987.984734666;-0.000225 2.38147015052435e-09 481864.819156963 -625615.408088608;-0.00015 2.3267887384569e-09 499358.724976525 -611742.72405756;-7.5e-05 2.27024732707299e-09 516453.451071785 -597381.022252878]  x3=[-0.000675 1.34333057909832e-11 1409.06764659014 -5515.47701855001;-0.0006 1.44923474351165e-11 1564.42956176314 -5473.43717855141;-0.000525 1.55398041184506e-11 1718.54089588104 -5427.02195661868;-0.00045 1.65748385201393e-11 1871.27845470133 -5376.26845637004;-0.000375 1.75966232495186e-11 2022.52014215645 -5321.21724937704;-0.0003 1.86043415075096e-11 2172.14505795553 -5261.91234273225;-0.000225 1.95971877395554e-11 2320.03359423021 -5198.40114387064;-0.00015 2.05743682795693e-11 2466.06753114737 -5130.73442267282;-7.5e-05 2.15351019843789e-11 2610.13013141223 -5058.96627088039]  x4=[-0.000675 -6.1472315632725e-12 5928.29142347644 -10182.4197288315;-0.0006 -7.25860860018538e-12 6213.78510946829 -10010.7531725388;-0.000525 -8.3641832164437e-12 6494.31159071774 -9831.08417332959;-0.00045 -9.4630716326151e-12 6769.64661864785 -9643.55635585287;-0.000375 -1.05543954141132e-11 7039.57009465009 -9448.31962697664;-0.0003 -1.1637282173405e-11 7303.86624602771 -9245.53005595474;-0.000225 -1.27108662673837e-11 7562.32379848114 -9035.34974966746;-0.00015 -1.37742894893511e-11 7814.73614499751 -8817.94672303579;-7.5e-05 -1.48267017550544e-11 8060.90151100904 -8593.49476471283]  x5=0.000667339049054976  V1=ones(3,3)  V2=ones(3,3)  I1=ones(3,3)  I2=ones(3,3)  nHarmo=1  Measurements=None  Decoupling=off  VsMag0=[ 1 1 1]  VrMag0=[ 1 1 1]  VsAngle0=[0 -120 120]  VrAngle0=[0 -120 120]  IsMag0=[ 1 1 1]  IrMag0=[ 1 1 1]  IsAngle0=[0 -120 120]  IrAngle0=[0 -120 120]
      settings: AttributesFormatString=\n  LibrarySourceBlock=sps_lib/Power Grid Elements/Distributed Parameters Line
  LMO 330 Mvar : spsThreePhaseSeriesRLCLoadLib/Three-Phase Series RLC Load  LConnTagsString=A|B|C  Configuration=Y (grounded)  NominalVoltage=735e3  Vabc=[1e3 1e3 1e3]  Vabcp=[1e3 1e3 1e3]  NominalFrequency=60  UnbalancedPower=off  ActivePower=1100000  InductivePower=330e6  CapacitivePower=0  Pabc=[10e3 9e3 11e3]  QLabc=[100 90 110]  QCabc=[100 90 110]  Pabcp=[10e3 9e3 11e3]  QLabcp=[100 90 110]  QCabcp=[100 90 110]  Measurements=None  LoadType=constant Z
  LMO-ALB 3*218km : spsDistributedParametersLineLib/Distributed Parameters Line  Phases=3  Length=218  Frequency=60  Resistance="[0.01273  0.3864]/3"  Inductance="[0.9337e-3  4.1264e-3]/3"  Capacitance=[12.74e-9 7.751e-9]*3  x1=[-0.001275 2.93013830402033e-09 0 0;-0.0012 2.90535199217008e-09 0 0;-0.001125 2.87824318639066e-09 0 0;-0.00105 2.84883355704664e-09 0 0;-0.000975 2.81714661374573e-09 0 0;-0.0009 2.78320768654558e-09 0 0;-0.000825 2.74704390570531e-09 329282.961098539 -717747.524634667;-0.00075 2.70868417999801e-09 349442.47113755 -708151.592396564;-0.000675 2.66815917360147e-09 369322.642211784 -697989.574610583;-0.0006 2.62550128158576e-09 388907.582416659 -687269.594638257;-0.000525 2.58074460401706e-09 408181.635850635 -676000.221867554;-0.00045 2.53392491869863e-09 427129.395130302 -664190.464862641;-0.000375 2.48507965257055e-09 445735.713706799 -651849.764162571;-0.0003 2.43424785179119e-09 463985.717973745 -638987.984734666;-0.000225 2.38147015052435e-09 481864.819156963 -625615.408088608;-0.00015 2.3267887384569e-09 499358.724976525 -611742.72405756;-7.5e-05 2.27024732707299e-09 516453.451071785 -597381.022252878]  x2=[-0.001275 9.46596966104073e-09 0 0;-0.0012 9.41521851949006e-09 0 0;-0.001125 9.35694099631258e-09 0 0;-0.00105 9.29118367766865e-09 0 0;-0.000975 9.21799912895266e-09 0 0;-0.0009 9.13744585277311e-09 0 0;-0.000825 9.04958824218646e-09 208359.206060548 -779372.311347812;-0.00075 8.95449652922236e-09 230309.218727174 -773170.335952688;-0.000675 8.85224672874118e-09 252075.125728199 -766350.300020907;-0.0006 8.74292057766896e-09 273639.527730595 -758917.655384841;-0.000525 8.62660546965812e-09 294985.186481349 -750878.343586891;-0.00045 8.50339438522633e-09 316095.038587454 -742238.791129901;-0.000375 8.37338581742929e-09 336952.209156129 -733005.904339916;-0.0003 8.23668369312689e-09 357540.025284346 -723187.063845369;-0.000225 8.0933972899057e-09 377842.029386896 -712790.118677116;-0.00015 7.94364114872408e-09 397841.992352332 -701823.379994047;-7.5e-05 7.78753498234996e-09 417523.926516267 -690295.61443927]  x3=[-0.001275 2.97611984430568e-11 0 0;-0.0012 3.12589199863691e-11 0 0;-0.001125 3.27316536273219e-11 0 0;-0.00105 3.4178222085176e-11 0 0;-0.000975 3.55974689952396e-11 0 0;-0.0009 3.69882598332479e-11 0 0;-0.000825 3.83494828222849e-11 -103.698287434019 -3735.86307129879;-0.00075 3.96800498215206e-11 1.95817417182707 -3737.30097845784;-0.000675 4.0978897196054e-11 107.613070443201 -3735.75134439733;-0.0006 4.2244986667167e-11 213.181942472598 -3731.21540787102;-0.000525 4.34773061423083e-11 318.580400118975 -3723.69679483717;-0.00045 4.46748705241445e-11 423.724189467941 -3713.20151556;-0.000375 4.58367224980322e-11 528.529260183044 -3699.73795980518;-0.0003 4.69619332972803e-11 632.911832694325 -3683.31689013319;-0.000225 4.80496034455922e-11 736.788465170426 -3663.95143329585;-0.00015 4.90988634760933e-11 840.076120220711 -3641.65706974308;-7.5e-05 5.01088746263694e-11 942.692231274088 -3616.45162124798]  x4=[-0.001275 1.84546523538988e-11 0 0;-0.0012 1.71318247858871e-11 0 0;-0.001125 1.57953022992672e-11 0 0;-0.00105 1.44461532896656e-11 0 0;-0.000975 1.30854562461578e-11 0 0;-0.0009 1.17142988891409e-11 0 0;-0.000825 1.03337773008269e-11 3660.66083936846 -13572.4875623715;-0.00075 8.94499504905071e-12 4042.89932356856 -13463.5735253587;-0.000675 7.5490623050953e-12 4421.90597590783 -13343.8969136693;-0.0006 6.14709495623774e-12 4797.3778242674 -13213.5533949555;-0.000525 4.74021371372586e-12 5169.01472219658 -13072.647163832;-0.00045 3.32954321689893e-12 5536.51958884542 -12921.2908585839;-0.000375 1.91621113416813e-12 5899.59864644653 -12759.6054711258;-0.0003 5.01347261575693e-13 6257.96165515655 -12587.7202502826;-0.000225 -9.13917380346779e-13 6611.32214506947 -12405.77259847;-0.00015 -2.32845145069881e-12 6959.39764521624 -12213.9079618568;-7.5e-05 -3.74112419258765e-12 7301.90990936778 -12012.2797140979]  x5=0.00123288061605072  V1=ones(3,3)  V2=ones(3,3)  I1=ones(3,3)  I2=ones(3,3)  nHarmo=1  Measurements=None  Decoupling=off  VsMag0=[ 1 1 1]  VrMag0=[ 1 1 1]  VsAngle0=[0 -120 120]  VrAngle0=[0 -120 120]  IsMag0=[ 1 1 1]  IrMag0=[ 1 1 1]  IsAngle0=[0 -120 120]  IrAngle0=[0 -120 120]
      settings: AttributesFormatString=\n  LibrarySourceBlock=sps_lib/Power Grid Elements/Distributed Parameters Line
  LMO7 : spsThreePhaseVIMeasurementLib/Three-Phase V-I Measurement  VoltageMeasurement=no  SetLabelV=on  LabelV=Vabc_LMO7  Vpu=on  VpuLL=off  CurrentMeasurement=no  SetLabelI=off  LabelI=A1  Ipu=off  Pbase=100e6  Vbase=735e3  OutputType=Magnitude  PhasorSimulation=off  PSBequivalent=0
  LVD 990 Mvar : spsThreePhaseSeriesRLCLoadLib/Three-Phase Series RLC Load  LConnTagsString=A|B|C  Configuration=Y (grounded)  NominalVoltage=735e3  Vabc=[1e3 1e3 1e3]  Vabcp=[1e3 1e3 1e3]  NominalFrequency=60  UnbalancedPower=off  ActivePower=3300000  InductivePower=990e6  CapacitivePower=0  Pabc=[10e3 9e3 11e3]  QLabc=[100 90 110]  QCabc=[100 90 110]  Pabcp=[10e3 9e3 11e3]  QLabcp=[100 90 110]  QCabcp=[100 90 110]  Measurements=None  LoadType=constant Z
  LVD-MTL 3*260km : spsDistributedParametersLineLib/Distributed Parameters Line  Phases=3  Length=260  Frequency=60  Resistance="[0.01273  0.3864]/3"  Inductance="[0.9337e-3  4.1264e-3]/3"  Capacitance=[12.74e-9 7.751e-9]*3  x1=[-0.0015 3.27622542096748e-08 -149994.752694911 -815900.545010622;-0.001425 3.26655309152711e-08 -126868.831368495 -819814.854171537;-0.00135 3.25426952952531e-08 -103641.493039442 -823073.815881615;-0.001275 3.23938455425361e-08 -80331.3052866202 -825674.824976729;-0.0012 3.22191006453347e-08 -56956.9019174628 -827615.802250005;-0.001125 3.20186002920463e-08 -33536.9680723824 -828895.196113909;-0.00105 3.17925047595854e-08 -10090.2252881576 -829511.983840561;-0.000975 3.15409947852613e-08 13364.5834677767 -829465.67237929;-0.0009 3.12642714222993e-08 36808.7087801719 -828756.298750769;-0.000825 3.09625558791217e-08 60223.4097739604 -827384.430017423;-0.00075 3.06360893425174e-08 83589.9690954246 -825351.162830128;-0.000675 3.02851327848405e-08 106889.707874563 -822658.122551563;-0.0006 2.99099667553934e-08 130104.000656695 -819307.461956921;-0.000525 2.951089115616e-08 153214.290291359 -815301.859513016;-0.00045 2.90882250020681e-08 176202.102766621 -810644.517237153;-0.000375 2.86423061659743e-08 199049.061976915 -805339.158137487;-0.0003 2.81734911085734e-08 221736.904412617 -799390.023236908;-0.000225 2.76821545934492e-08 244247.49375962 -792801.868182831;-0.00015 2.71686893874941e-08 266562.835397223 -785579.959445605;-7.5e-05 2.66335059469376e-08 288665.090782758 -777730.070108574]  x2=[-0.0015 4.84558088676577e-08 -353353.509255419 -707507.476279917;-0.001425 4.82587092400841e-08 -333210.629182316 -717214.190537853;-0.00135 4.80230323387271e-08 -312801.385630537 -726347.574745618;-0.001275 4.77489665600955e-08 -292142.093437108 -734900.327815623;-0.0012 4.74367309881795e-08 -271249.267324108 -742865.612807923;-0.001125 4.70865752193179e-08 -250139.608697063 -750237.06239557;-0.00105 4.66987791626746e-08 -228829.99229409 -757008.78395455;-0.000975 4.62736528164841e-08 -207337.452696493 -763175.36427426;-0.0009 4.58115360202426e-08 -185679.17071158 -768731.873884743;-0.000825 4.53127981830466e-08 -163872.459638586 -773673.870997235;-0.00075 4.47778379882921e-08 -141934.751428691 -777997.405054859;-0.000675 4.42070830749737e-08 -119883.582750177 -781699.019890641;-0.0006 4.36009896958362e-08 -97736.5809698939 -784775.756490319;-0.000525 4.29600423526533e-08 -75511.4500622029 -787225.155357731;-0.00045 4.22847534089244e-08 -53225.9564566961 -789045.258480898;-0.000375 4.15756626802989e-08 -30897.9148359823 -790234.610897233;-0.0003 4.08333370030557e-08 -8545.17389490259 -790792.261856611;-0.000225 4.00583697809833e-08 13814.3979274432 -790717.765581389;-0.00015 3.92513805110215e-08 36162.9267314532 -790011.181622749;-7.5e-05 3.84130142880455e-08 58482.5474451453 -788673.074813096]  x3=[-0.0015 1.7587712979714e-10 176.513539924873 -1804.55713842236;-0.001425 1.79321128612803e-10 227.459268206894 -1798.84517601097;-0.00135 1.82621780861958e-10 278.223169030154 -1791.69524428912;-0.001275 1.85776448053699e-10 328.764662509049 -1783.11305880285;-0.0012 1.88782608395341e-10 379.043346547001 -1773.10548001992;-0.001125 1.91637858808303e-10 429.019029133282 -1761.68050784568;-0.00105 1.9433991684909e-10 478.651760471885 -1748.84727522809;-0.000975 1.96886622533849e-10 527.901864916785 -1734.61604085694;-0.0009 1.99275940065021e-10 576.729972688039 -1718.99818096324;-0.000825 2.01505959458729e-10 625.097051343391 -1702.00618022524;-0.00075 2.0357489807159e-10 672.964436980204 -1683.65362178833;-0.000675 2.05481102025733e-10 720.293865142797 -1663.95517640693;-0.0006 2.07223047530883e-10 767.04750141046 -1642.92659071687;-0.000525 2.08799342102456e-10 813.187971641716 -1620.58467464782;-0.00045 2.10208725674689e-10 858.678391850635 -1596.94728798563;-0.000375 2.11450071607919e-10 903.482397691328 -1572.03332609554;-0.0003 2.12522387589201e-10 947.564173527052 -1545.86270481748;-0.000225 2.13424816425545e-10 990.888481060676 -1518.45634454569;-0.00015 2.14156636729147e-10 1033.42068750364 -1489.83615350522;-7.5e-05 2.14717263494055e-10 1075.12679326088 -1460.02501023891]  x4=[-0.0015 1.36498831241419e-10 -8566.49009753062 -13975.61804386;-0.001425 1.34439683009913e-10 -8167.96786665097 -14212.2119177605;-0.00135 1.32273065752805e-10 -7762.91628723282 -14437.444766908;-0.001275 1.3000071143078e-10 -7351.65915131126 -14651.1365436092;-0.0012 1.27624436529115e-10 -6934.5252115483 -14853.1164259273;-0.001125 1.25146140605608e-10 -6511.84791843301 -15043.2229542348;-0.00105 1.22567804772101e-10 -6083.96515372635 -15221.3041602818;-0.000975 1.1989149011081e-10 -5651.21896036359 -15387.2176886767;-0.0009 1.17119336026725e-10 -5213.95526903046 -15540.8309106837;-0.000825 1.14253558537407e-10 -4772.52362163146 -15682.0210302434;-0.00075 1.11296448501531e-10 -4327.27689187139 -15810.6751821344;-0.000675 1.08250369787617e-10 -3878.57100317351 -15926.6905221963;-0.0006 1.0511775738438e-10 -3426.76464415983 -16029.9743095413;-0.000525 1.01901115454246e-10 -2972.21898192085 -16120.4439806901;-0.00045 9.86030153315568e-11 -2515.29737330421 -16198.0272155717;-0.000375 9.52260934670886e-11 -2056.36507445269 -16262.6619953354;-0.0003 9.17730493205108e-11 -1595.78894882409 -16314.2966519271;-0.000225 8.8246643202481e-11 -1133.93717392619 -16352.8899093923;-0.00015 8.4649694068094e-11 -671.178947001271 -16378.4109168716;-7.5e-05 8.09850772634528e-11 -207.884189895504 -16390.839273262]  x5=0.00147040807418893  V1=ones(3,3)  V2=ones(3,3)  I1=ones(3,3)  I2=ones(3,3)  nHarmo=1  Measurements=None  Decoupling=off  VsMag0=[ 1 1 1]  VrMag0=[ 1 1 1]  VsAngle0=[0 -120 120]  VrAngle0=[0 -120 120]  IsMag0=[ 1 1 1]  IrMag0=[ 1 1 1]  IsAngle0=[0 -120 120]  IrAngle0=[0 -120 120]
      settings: AttributesFormatString=\n  LibrarySourceBlock=sps_lib/Power Grid Elements/Distributed Parameters Line
  LVD7 : spsThreePhaseVIMeasurementLib/Three-Phase V-I Measurement  VoltageMeasurement=no  SetLabelV=on  LabelV=Vabc_LVD7  Vpu=on  VpuLL=off  CurrentMeasurement=no  SetLabelI=off  LabelI=A1  Ipu=off  Pbase=100e6  Vbase=735e3  OutputType=Magnitude  PhasorSimulation=off  PSBequivalent=0
  Load Flow Bus1 : spsLoadFlowBusLib/Load Flow Bus  LConnTagsString=a  Phases=single  Connectors=on one side  ID=LG31_13.8  Vbase=13.8e3  Vref=1  Vangle=0  VLF=1  VLFb=1  VLFc=1  angleLF=-0.0351  angleLFb=0  angleLFc=0
      settings: AttributesFormatString=%<ID>\n%<Vbase>V\n%<VLF>pu\n%<angleLF>deg.
  Load Flow Bus10 : spsLoadFlowBusLib/Load Flow Bus  LConnTagsString=a  Phases=single  Connectors=on one side  ID=LVD7  Vbase=735e3  Vref=1  Vangle=0  VLF=1.05  VLFb=1  VLFc=1  angleLF=-12.02  angleLFb=0  angleLFc=0
      settings: AttributesFormatString=%<ID>\n%<Vbase>V\n%<VLF>pu\n%<angleLF>deg.
  Load Flow Bus11 : spsLoadFlowBusLib/Load Flow Bus  LConnTagsString=a  Phases=single  Connectors=on one side  ID=CHM7  Vbase=735e3  Vref=1  Vangle=0  VLF=1.047  VLFb=1  VLFc=1  angleLF=-4.064  angleLFb=0  angleLFc=0
      settings: AttributesFormatString=%<ID>\n%<Vbase>V\n%<VLF>pu\n%<angleLF>deg.
  Load Flow Bus12 : spsLoadFlowBusLib/Load Flow Bus  LConnTagsString=a  Phases=single  Connectors=on one side  ID=LG47  Vbase=735e3  Vref=1  Vangle=0  VLF=1.004  VLFb=1  VLFc=1  angleLF=20.71  angleLFb=0  angleLFc=0
      settings: AttributesFormatString=%<ID>\n%<Vbase>V\n%<VLF>pu\n%<angleLF>deg.
  Load Flow Bus2 : spsLoadFlowBusLib/Load Flow Bus  LConnTagsString=a  Phases=single  Connectors=on one side  ID=LG3_13.8  Vbase=13.8e3  Vref=1  Vangle=0  VLF=1  VLFb=1  VLFc=1  angleLF=-0.6025  angleLFb=0  angleLFc=0
      settings: AttributesFormatString=%<ID>\n%<Vbase>V\n%<VLF>pu\n%<angleLF>deg.
  Load Flow Bus3 : spsLoadFlowBusLib/Load Flow Bus  LConnTagsString=a  Phases=single  Connectors=on one side  ID=LG4_13.8  Vbase=13.8e3  Vref=1  Vangle=0  VLF=1  VLFb=1  VLFc=1  angleLF=-3.293  angleLFb=0  angleLFc=0
      settings: AttributesFormatString=%<ID>\n%<Vbase>V\n%<VLF>pu\n%<angleLF>deg.
  Load Flow Bus4 : spsLoadFlowBusLib/Load Flow Bus  LConnTagsString=a  Phases=single  Connectors=on one side  ID=LG2_13.8  Vbase=13.8e3  Vref=1  Vangle=0  VLF=1  VLFb=1  VLFc=1  angleLF=0  angleLFb=0  angleLFc=0
      settings: AttributesFormatString=%<ID>\n%<Vbase>V\n%<VLF>pu\n%<angleLF>deg.
  Load Flow Bus5 : spsLoadFlowBusLib/Load Flow Bus  LConnTagsString=a  Phases=single  Connectors=on one side  ID=LG27  Vbase=735e3  Vref=1  Vangle=0  VLF=1  VLFb=1  VLFc=1  angleLF=23.57  angleLFb=0  angleLFc=0
      settings: AttributesFormatString=%<ID>\n%<Vbase>V\n%<VLF>pu\n%<angleLF>deg.
  Load Flow Bus6 : spsLoadFlowBusLib/Load Flow Bus  LConnTagsString=a  Phases=single  Connectors=on one side  ID=LG37  Vbase=735e3  Vref=1  Vangle=0  VLF=0.994  VLFb=1  VLFc=1  angleLF=24.1  angleLFb=0  angleLFc=0
      settings: AttributesFormatString=%<ID>\n%<Vbase>V\n%<VLF>pu\n%<angleLF>deg.
  Load Flow Bus7 : spsLoadFlowBusLib/Load Flow Bus  LConnTagsString=a  Phases=single  Connectors=on one side  ID=LMO7  Vbase=735e3  Vref=1  Vangle=0  VLF=1.016  VLFb=1  VLFc=1  angleLF=17.31  angleLFb=0  angleLFc=0
      settings: AttributesFormatString=%<ID>\n%<Vbase>V\n%<VLF>pu\n%<angleLF>deg.
  Load Flow Bus8 : spsLoadFlowBusLib/Load Flow Bus  LConnTagsString=a  Phases=single  Connectors=on one side  ID=NEM_ALB7  Vbase=735e3  Vref=1  Vangle=0  VLF=1.028  VLFb=1  VLFc=1  angleLF=8.928  angleLFb=0  angleLFc=0
      settings: AttributesFormatString=%<ID>\n%<Vbase>V\n%<VLF>pu\n%<angleLF>deg.
  Load Flow Bus9 : spsLoadFlowBusLib/Load Flow Bus  LConnTagsString=a  Phases=single  Connectors=on one side  ID=ABI_CHB7  Vbase=735e3  Vref=1  Vangle=0  VLF=1.046  VLFb=1  VLFc=1  angleLF=0.1334  angleLFb=0  angleLFc=0
      settings: AttributesFormatString=%<ID>\n%<Vbase>V\n%<VLF>pu\n%<angleLF>deg.
  NEM-ABI 6*236 : spsDistributedParametersLineLib/Distributed Parameters Line  Phases=3  Length=236  Frequency=60  Resistance="[0.01273  0.3864]/6"  Inductance="[0.9337e-3  4.1264e-3]/6"  Capacitance=[12.74e-9 7.751e-9]*6  x1=[-0.00135 9.63678145672075e-09 0 0;-0.001275 9.58707971475536e-09 0 0;-0.0012 9.52971420795322e-09 0 0;-0.001125 9.46473079342277e-09 0 0;-0.00105 9.39218141791129e-09 0 0;-0.000975 9.31212407627953e-09 0 0;-0.0009 9.22462276514147e-09 0 0;-0.000825 9.12974743170642e-09 235173.136251889 -772031.417007134;-0.00075 9.02757391786428e-09 256904.899781863 -765074.329412112;-0.000675 8.91818389955871e-09 278431.297465728 -757505.653104188;-0.0006 8.80166482149662e-09 299735.12143054 -749331.438367397;-0.000525 8.67810982724622e-09 320799.341725382 -740558.219543931;-0.00045 8.54761768477945e-09 341607.119934843 -731193.009810682;-0.000375 8.41029270751839e-09 362141.822639392 -721243.295573019;-0.0003 8.26624467094875e-09 382387.03471188 -710717.030480267;-0.000225 8.11558872486694e-09 402326.572439536 -699622.629067684;-0.00015 7.95844530133113e-09 421944.496460987 -687968.96003001;-7.5e-05 7.79494001838974e-09 441225.124507935 -675765.339131966]  x2=[-0.00135 1.61909577854842e-08 0 0;-0.001275 1.61138836815729e-08 0 0;-0.0012 1.60239283855973e-08 0 0;-0.001125 1.59211638064445e-08 0 0;-0.00105 1.58056720925469e-08 0 0;-0.000975 1.56775455662134e-08 0 0;-0.0009 1.55368866498287e-08 0 0;-0.000825 1.53838077839785e-08 81706.5138318975 -820341.45742731;-0.00075 1.52184313375659e-08 104865.377019311 -817703.667465169;-0.000675 1.50408895099919e-08 127940.412428829 -814412.217702543;-0.0006 1.48513242254769e-08 150913.174230206 -810469.739274009;-0.000525 1.46498870196089e-08 173765.298349152 -805879.383736503;-0.00045 1.44367389182083e-08 196478.517147295 -800644.820550007;-0.000375 1.4212050308606e-08 219034.674025054 -794770.234144239;-0.0003 1.39760008034386e-08 241415.73793574 -788260.320573688;-0.000225 1.3728779097069e-08 263603.817799304 -781120.283763658;-0.00015 1.34705828147465e-08 285581.176804193 -773355.831350329;-7.5e-05 1.32016183546287e-08 307330.246585884 -764973.170118159]  x3=[-0.00135 1.11391405873975e-10 0 0;-0.001275 1.14303695093123e-10 0 0;-0.0012 1.17124611687319e-10 0 0;-0.001125 1.19851900658998e-10 0 0;-0.00105 1.22483381855087e-10 0 0;-0.000975 1.25016951709778e-10 0 0;-0.0009 1.27450584926097e-10 0 0;-0.000825 1.29782336094885e-10 -1379.76964293888 -6710.39772289696;-0.00075 1.32010341249935e-10 -1189.51028635481 -6746.72121820831;-0.000675 1.34132819358016e-10 -998.300053447941 -6777.65148780611;-0.0006 1.36148073742603e-10 -806.291794752853 -6803.16380650611;-0.000525 1.38054493440175e-10 -613.638998733716 -6823.23778015108;-0.00045 1.39850554487996e-10 -420.495669087984 -6837.85736191364;-0.000375 1.41534821142345e-10 -227.016201638182 -6847.01086512381;-0.0003 1.43105947026228e-10 -33.3552609102555 -6850.69097261118;-0.000225 1.44562676205652e-10 160.33234350289 -6848.89474255413;-0.00015 1.45903844193601e-10 353.891780693807 -6841.62361083148;-7.5e-05 1.47128378880905e-10 547.168322209963 -6828.88338987469]  x4=[-0.00135 9.42674768711692e-11 0 0;-0.001275 9.17338278957505e-11 0 0;-0.0012 8.91268483018866e-11 0 0;-0.001125 8.64486220691766e-11 0 0;-0.00105 8.37012901306928e-11 0 0;-0.000975 8.08870486615512e-11 0 0;-0.0009 7.80081473233229e-11 0 0;-0.000825 7.5066887465689e-11 2916.74328192385 -29367.0114377977;-0.00075 7.2065620286777e-11 3745.79818278167 -29272.8158501724;-0.000675 6.90067449536486e-11 4571.85874988483 -29155.2200214456;-0.0006 6.5892706684443e-11 5394.2646430551 -29014.3179559235;-0.000525 6.2725994793706e-11 6212.35844360473 -28850.2222885613;-0.00045 5.95091407024708e-11 7025.48617986682 -28663.0641949249;-0.000375 5.62447159146784e-11 7832.99784997026 -28452.9932863306;-0.0003 5.29353299615569e-11 8634.24794144133 -28220.1774902486;-0.000225 4.95836283156018e-11 9428.59594721643 -27964.8029160642;-0.00015 4.61922902758261e-11 10215.4068776537 -27687.0737063044;-7.5e-05 4.27640268259697e-11 10994.0517681339 -27387.2118734503]  x5=0.00133467809810995  V1=ones(3,3)  V2=ones(3,3)  I1=ones(3,3)  I2=ones(3,3)  nHarmo=1  Measurements=None  Decoupling=off  VsMag0=[ 1 1 1]  VrMag0=[ 1 1 1]  VsAngle0=[0 -120 120]  VrAngle0=[0 -120 120]  IsMag0=[ 1 1 1]  IrMag0=[ 1 1 1]  IsAngle0=[0 -120 120]  IrAngle0=[0 -120 120]
      settings: AttributesFormatString=\n  LibrarySourceBlock=sps_lib/Power Grid Elements/Distributed Parameters Line
  NEM-ALB 1980 Mvar : spsThreePhaseSeriesRLCLoadLib/Three-Phase Series RLC Load  LConnTagsString=A|B|C  Configuration=Y (grounded)  NominalVoltage=735e3  Vabc=[1e3 1e3 1e3]  Vabcp=[1e3 1e3 1e3]  NominalFrequency=60  UnbalancedPower=off  ActivePower=6600000  InductivePower=1980e6  CapacitivePower=0  Pabc=[10e3 9e3 11e3]  QLabc=[100 90 110]  QCabc=[100 90 110]  Pabcp=[10e3 9e3 11e3]  QLabcp=[100 90 110]  QCabcp=[100 90 110]  Measurements=None  LoadType=constant Z
  NEM-ALB7 : spsThreePhaseVIMeasurementLib/Three-Phase V-I Measurement  VoltageMeasurement=no  SetLabelV=on  LabelV=Vabc_NEM7  Vpu=on  VpuLL=off  CurrentMeasurement=no  SetLabelI=off  LabelI=A1  Ipu=off  Pbase=100e6  Vbase=735e3  OutputType=Magnitude  PhasorSimulation=off  PSBequivalent=0
  Regulators1 : Subsystem
  Regulators2 : Subsystem
  Regulators3 : Subsystem
  Regulators4 : Subsystem
  MTLa : PMIOPort  Side=Right
  MTLb : PMIOPort  Port=2  Side=Right
  MTLc : PMIOPort  Port=3  Side=Right
  CHM7a : PMIOPort  Port=4  Side=Right
  CHM7b : PMIOPort  Port=5  Side=Right
  CHM7c : PMIOPort  Port=6  Side=Right
  wires:
  Regulators2/1(Pm) -> LG3_2200 MVA/1
  Regulators4/2(Vf) -> LG4-2700 MVA/2
  Regulators4/1(Pm) -> LG4-2700 MVA/1
  Regulators3/2(Vf) -> LG31-200 MVA/2
  Regulators3/1(Pm) -> LG31-200 MVA/1
  Regulators2/2(Vf) -> LG3_2200 MVA/2
  LG3_2200 MVA/1 -> Regulators2/1(m)
  Regulators1/1(Pm) -> LG2_5500 MVA/1
  Regulators1/2(Vf) -> LG2_5500 MVA/2
  LG2_5500 MVA/1 -> Regulators1/1(m)
  LG31-200 MVA/1 -> Regulators3/1(m)
  LG4-2700 MVA/1 -> Regulators4/1(m)
  connections:
  LG2-NENI 3*279km/RConn1 -- "Cs NEM "/LConn1
  LG2-NENI 3*279km/RConn2 -- "Cs NEM "/LConn2
  LG2-NENI 3*279km/RConn3 -- "Cs NEM "/LConn3
  CHB-CHM 3*195km/RConn1 -- "Cs  CHMN "/LConn1
  CHB-CHM 3*195km/RConn2 -- "Cs  CHMN "/LConn2
  CHB-CHM 3*195km/RConn3 -- "Cs  CHMN "/LConn3
  Load Flow Bus2/LConn1 -- 2200 MVA 13.8 kV/735 kV/LConn1 -- LG3_2200 MVA/RConn1 -- 110 MW/LConn1
  2200 MVA 13.8 kV/735 kV/LConn2 -- LG3_2200 MVA/RConn2 -- 110 MW/LConn2
  2200 MVA 13.8 kV/735 kV/LConn3 -- LG3_2200 MVA/RConn3 -- 110 MW/LConn3
  Load Flow Bus1/LConn1 -- 200 MVA 13.8 kV/735 kV/LConn1 -- LG31-200 MVA/RConn1 -- 10 MW/LConn1
  200 MVA 13.8 kV/735 kV/LConn2 -- LG31-200 MVA/RConn2 -- 10 MW/LConn2
  200 MVA 13.8 kV/735 kV/LConn3 -- LG31-200 MVA/RConn3 -- 10 MW/LConn3
  Load Flow Bus6/LConn1 -- 2200 MVA 13.8 kV/735 kV/RConn1 -- 200 MVA 13.8 kV/735 kV/RConn1 -- LG3-LMO 104km/LConn1 -- LG3 660 Mvar/LConn1 -- LG2-LG3 155km/RConn1
  2200 MVA 13.8 kV/735 kV/RConn2 -- LG3 660 Mvar/LConn2 -- LG2-LG3 155km/RConn2 -- 200 MVA 13.8 kV/735 kV/RConn2 -- LG3-LMO 104km/LConn2
  LG3-LMO 104km/RConn1 -- LMO7/RConn1 -- LG4-LMO 3*118km/RConn1 -- LMO 330 Mvar/LConn1
  LG3-LMO 104km/RConn2 -- LMO7/RConn2 -- LG4-LMO 3*118km/RConn2 -- LMO 330 Mvar/LConn2
  LG3-LMO 104km/RConn3 -- LMO7/RConn3 -- LG4-LMO 3*118km/RConn3 -- LMO 330 Mvar/LConn3
  LG4-LMO 3*118km/LConn1 -- LG4 660 Mvar/LConn1 -- 2700 MVA 13.8 kV/735 kV/RConn1 -- Load Flow Bus12/LConn1
  LG4-LMO 3*118km/LConn2 -- 2700 MVA 13.8 kV/735 kV/RConn2 -- LG4 660 Mvar/LConn2
  LG4 660 Mvar/LConn3 -- 2700 MVA 13.8 kV/735 kV/RConn3 -- LG4-LMO 3*118km/LConn3
  Load Flow Bus3/LConn1 -- LG4-2700 MVA/RConn1 -- 2700 MVA 13.8 kV/735 kV/LConn1 -- 135 MW/LConn1
  LG4-2700 MVA/RConn2 -- 2700 MVA 13.8 kV/735 kV/LConn2 -- 135 MW/LConn2
  LG4-2700 MVA/RConn3 -- 2700 MVA 13.8 kV/735 kV/LConn3 -- 135 MW/LConn3
  Load Flow Bus4/LConn1 -- 5500 MVA 13.8 kV/735 kV/LConn1 -- LG2_5500 MVA/RConn1 -- 275 MW/LConn1
  5500 MVA 13.8 kV/735 kV/LConn2 -- LG2_5500 MVA/RConn2 -- 275 MW/LConn2
  LG2_5500 MVA/RConn3 -- 5500 MVA 13.8 kV/735 kV/LConn3 -- 275 MW/LConn3
  5500 MVA 13.8 kV/735 kV/RConn1 -- LG2-NENI 3*279km/LConn1 -- LG2-LG3 155km/LConn1 -- LG2 660 Mvar/LConn1 -- Load Flow Bus5/LConn1
  LG2-LG3 155km/LConn2 -- 5500 MVA 13.8 kV/735 kV/RConn2 -- LG2-NENI 3*279km/LConn2 -- LG2 660 Mvar/LConn2
  LG2-LG3 155km/LConn3 -- 5500 MVA 13.8 kV/735 kV/RConn3 -- LG2-NENI 3*279km/LConn3 -- LG2 660 Mvar/LConn3
  "Cs NEM "/RConn1 -- NEM-ALB7/LConn1 -- Cs ALB/RConn1
  "Cs NEM "/RConn2 -- NEM-ALB7/LConn2 -- Cs ALB/RConn2
  "Cs NEM "/RConn3 -- NEM-ALB7/LConn3 -- Cs ALB/RConn3
  LMO7/LConn1 -- LMO-ALB 3*218km/LConn1
  LMO7/LConn2 -- LMO-ALB 3*218km/LConn2
  Load Flow Bus7/LConn1 -- LMO7/LConn3 -- LMO-ALB 3*218km/LConn3
  Cs ALB/LConn1 -- LMO-ALB 3*218km/RConn1
  Cs ALB/LConn2 -- LMO-ALB 3*218km/RConn2
  Cs ALB/LConn3 -- LMO-ALB 3*218km/RConn3
  200 MVA 13.8 kV/735 kV/RConn3 -- LG3-LMO 104km/LConn3 -- LG3 660 Mvar/LConn3 -- LG2-LG3 155km/RConn3 -- 2200 MVA 13.8 kV/735 kV/RConn3
  Load Flow Bus8/LConn1 -- NEM-ABI 6*236/LConn1 -- NEM-ALB7/RConn1 -- NEM-ALB 1980 Mvar/LConn1
  NEM-ALB 1980 Mvar/LConn2 -- NEM-ALB7/RConn2 -- NEM-ABI 6*236/LConn2
  NEM-ALB 1980 Mvar/LConn3 -- NEM-ALB7/RConn3 -- NEM-ABI 6*236/LConn3
  NEM-ABI 6*236/RConn1 -- "Cs ABI+CHB "/LConn1
  NEM-ABI 6*236/RConn2 -- "Cs ABI+CHB "/LConn2
  NEM-ABI 6*236/RConn3 -- "Cs ABI+CHB "/LConn3
  "Cs ABI+CHB "/RConn1 -- ABI-CHB7/LConn1
  "Cs ABI+CHB "/RConn2 -- ABI-CHB7/LConn2
  "Cs ABI+CHB "/RConn3 -- ABI-CHB7/LConn3
  Load Flow Bus9/LConn1 -- ABI+CHB 1320 Mvar/LConn1 -- CHB-CHM 3*195km/LConn1 -- ABI-CHB 3*271km/LConn1 -- ABI-CHB7/RConn1
  ABI-CHB 3*271km/LConn2 -- ABI-CHB7/RConn2 -- ABI+CHB 1320 Mvar/LConn2 -- CHB-CHM 3*195km/LConn2
  ABI-CHB 3*271km/LConn3 -- ABI-CHB7/RConn3 -- ABI+CHB 1320 Mvar/LConn3 -- CHB-CHM 3*195km/LConn3
  ABI-CHB 3*271km/RConn1 -- "Cs LVDN "/LConn1
  ABI-CHB 3*271km/RConn2 -- "Cs LVDN "/LConn2
  ABI-CHB 3*271km/RConn3 -- "Cs LVDN "/LConn3
  "Cs LVDN "/RConn1 -- LVD7/LConn1
  "Cs LVDN "/RConn2 -- LVD7/LConn2
  "Cs LVDN "/RConn3 -- LVD7/LConn3
  "Cs LVDS "/LConn1 -- LVD 990 Mvar/LConn1 -- Load Flow Bus10/LConn1 -- LVD7/RConn1
  "Cs LVDS "/LConn2 -- LVD7/RConn2 -- LVD 990 Mvar/LConn2
  "Cs LVDS "/LConn3 -- LVD7/RConn3 -- LVD 990 Mvar/LConn3
  "Cs LVDS "/RConn1 -- LVD-MTL 3*260km/LConn1
  "Cs LVDS "/RConn2 -- LVD-MTL 3*260km/LConn2
  "Cs LVDS "/RConn3 -- LVD-MTL 3*260km/LConn3
  MTLa/RConn1 -- LVD-MTL 3*260km/RConn1
  MTLb/RConn1 -- LVD-MTL 3*260km/RConn2
  MTLc/RConn1 -- LVD-MTL 3*260km/RConn3
  "Cs  CHMN "/RConn1 -- CHM7/LConn1
  "Cs  CHMN "/RConn2 -- CHM7/LConn2
  "Cs  CHMN "/RConn3 -- CHM7/LConn3
  CHM 1320Mvar/LConn2 -- CHM7/RConn2 -- CHM7b/RConn1
  Load Flow Bus11/LConn1 -- CHM 1320Mvar/LConn3 -- CHM7c/RConn1 -- CHM7/RConn3
  CHM7a/RConn1 -- CHM 1320Mvar/LConn1 -- CHM7/RConn1
